simulink model "Gel"  (R2015a)
settings: Solver=ode45  StartTime=0.0  StopTime=10e-3  RelTol=1e-3
undefined symbols (not defined in the file): KEL, L, RL
settings Model: DataDictionary=dataDict_galvoMod6860.sldd  Creator=mainster  LastModifiedBy=mainster

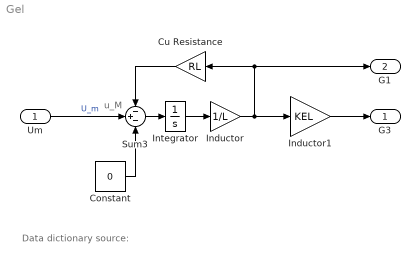
== system Gel ==
  note: u_M
  note: Data dictionary source:
  Um : Inport
  Constant : Constant  Value=0
  Cu Resistance : Gain  Gain=RL
  Inductor : Gain  Gain=1/L
  Inductor1 : Gain  Gain=KEL
  Integrator : Integrator
  Sum3 : Sum  Inputs=-+-
  G3 : Outport
  G1 : Outport  Port=2
  wires:
  Um/1 -> Sum3/2  "U_m"
  Sum3/1 -> Integrator/1
  Cu Resistance/1 -> Sum3/1
  Integrator/1 -> Inductor/1
  Inductor/1 -> Inductor1/1, Cu Resistance/1, G1/1
  Constant/1 -> Sum3/3
  Inductor1/1 -> G3/1
